simulink model "test"  (R2017a)
settings: Solver=VariableStepAuto  StartTime=0.0  StopTime=2  MaxStep=0.002  RelTol=1e-3
undefined symbols (not defined in the file): den, num
settings Model: Creator=JakobLab  LastModifiedBy=JakobLab

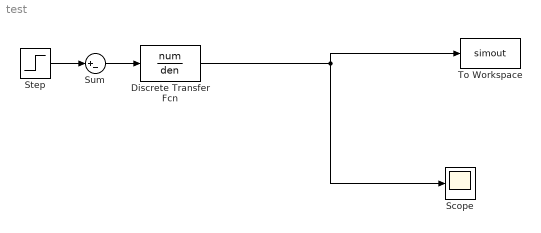
== system test ==
  Discrete Transfer Fcn : DiscreteTransferFcn  Numerator=num  Denominator=den
  Scope : Scope
  Step : Step  SampleTime=0
  Sum : Sum  Inputs=|+-
  To Workspace : ToWorkspace  VariableName=simout  SaveFormat=Structure With Time  SampleTime=-1
  wires:
  Discrete Transfer Fcn/1 -> Scope/1, To Workspace/1
  Step/1 -> Sum/1
  Sum/1 -> Discrete Transfer Fcn/1
